simulink model "QuickModel"  (R2023b)
settings: Solver=VariableStepAuto  StartTime=0.0  StopTime=10.0  RelTol=1e-3
model workspace (MAT data in the model file):
  pqr = [0 0 0]
values from neighbouring files (symbols this model uses):
  alpha1 = 2.6    [QuickModel.m]    (also in QuickModelCode.m)
  alphadot = 0    [QuickModel.m]    (also in QuickModelCode.m)
  c_D_1 = .030    (= 0.03)    [QuickModel.m]    (also in QuickModelCode.m)
  c_D_alpha = ((2*c_L_1)/(pi*AR*e))*c_L_alpha    [QuickModel.m]    (also in QuickModelCode.m)
  c_D_delta_E = 0    [QuickModel.m]    (also in QuickModelCode.m)
  c_D_q = 0    [QuickModel.m]    (also in QuickModelCode.m)
  c_D_u = 0    [QuickModel.m]    (also in QuickModelCode.m)
  c_L_1 = .26    (= 0.26)    [QuickModel.m]    (also in QuickModelCode.m)
  c_L_alpha = c_L_alpha_W_mach + c_L_alpha_H    [QuickModel.m]    (also in QuickModelCode.m)
  c_L_alphadot = 2*c_L_alpha_H_mach*eta_H*(S_H/S_ft2)*(xbar_AC_H - xbar_CG)*(d_epsilon_dalpha_mach)    [QuickModel.m]    (also in QuickModelCode.m)
  c_L_delta_E = 0    [QuickModel.m]    (also in QuickModelCode.m)
  c_L_i_H = c_L_alpha_H_mach*eta_H*(S_H/S_ft2)    [QuickModel.m]    (also in QuickModelCode.m)
  c_L_q = piece1+piece2+piece3    [QuickModel.m]    (also in QuickModelCode.m)
  c_L_u = ((Mach^2)/(1-Mach^2))*c_L_1    (= 1.10842105263)    [QuickModel.m]    (also in QuickModelCode.m)
  c_m_1 = 0    [QuickModel.m]    (also in QuickModelCode.m)
  c_m_alpha = (c_L_alpha_W_mach*(xbar_CG - xbar_AC_WB)) - c_L_alpha_H_mach*eta_H*(S_H/S_ft2)*(1-d_epsilon_dalpha_mach)*(xbar_AC_H - xbar_CG)    [QuickModel.m]    (also in QuickModelCode.m)
  c_m_alphadot = -2*c_L_alpha_H_mach*eta_H*(S_H/S_ft2)*((xbar_AC_H - xbar_CG)^2)*d_epsilon_dalpha_mach    [QuickModel.m]    (also in QuickModelCode.m)
  c_m_delta_E = c_m_i_H * tau_E    [QuickModel.m]    (also in QuickModelCode.m)
  c_m_i_H = -c_L_alpha_H_mach*eta_H*(S_H/S_ft2) * (xbar_AC_H - xbar_CG)    [QuickModel.m]    (also in QuickModelCode.m)
  c_m_q = (frac * secondpiece * thirdpiece) + fourthpiece    [QuickModel.m]    (also in QuickModelCode.m)
  cbar_ft = 16.0    (= 16)    [QuickModel.m]    (also in QuickModelCode.m)
  deltaA = 0    [QuickModel.m]    (also in QuickModelCode.m)
  deltaE = 0    [QuickModel.m]    (also in QuickModelCode.m)
  i_H = 0    [QuickModel.m]    (also in QuickModelCode.m)
  qbar1 = 283.2    [QuickModel.m]    (also in QuickModelCode.m)
  S_ft2 = 530    [QuickModel.m]    (also in QuickModelCode.m)
  uv = a*Mach    (= 871.2)    [QuickModel.m]    (also in QuickModelCode.m)
  V_P_1 = 0    [QuickModel.m]    (also in QuickModelCode.m)
undefined symbols (not defined in the file or in its folder): c_D_i_H, c_m_u, delta_Stabilitator
libraries: shared6dof x1
settings Model: Creator=Owner  LastModifiedBy=Owner

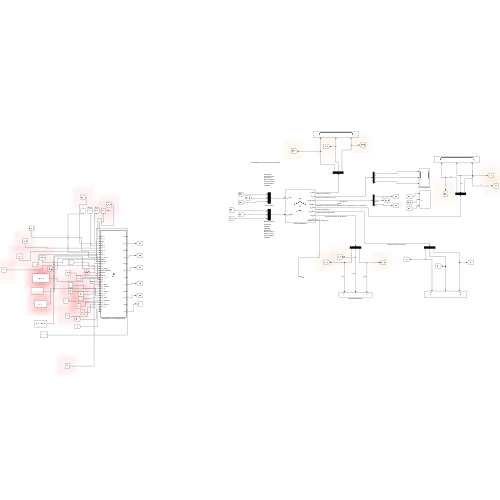
[thumbnail: Simulink's stored preview of the top-level diagram]
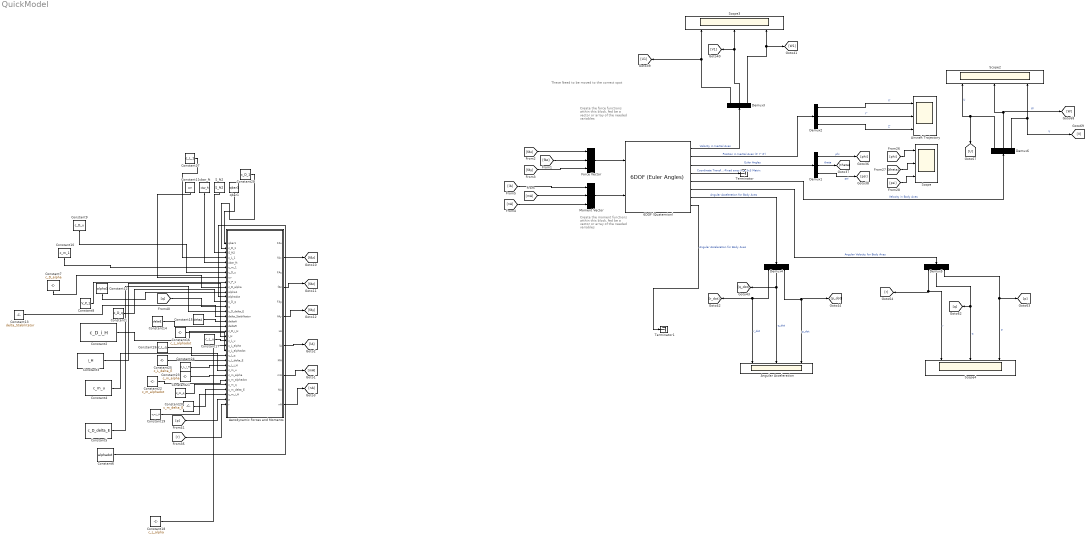
== system QuickModel ==
  note: These Need to be moved to the correct spot
  note: Create the moment functions within this block, fed be a vector or array of the needed variables
  note: Create the force functions within this block, fed be a vector or array of the needed variables
  6DOF (Quaternion) : shared6dof/6DOF (Euler Angles)  units=English (Velocity in ft/s)  mtype=Fixed  rep=Quaternion  xme_0=InitialInertialPosition  Vm_0=InitialVelocity  eul_0=InitialEulerOrientation  pm_0=pqr  mass_0=1.0  mass_e=0.5  mass_f=2.0  inertia=eye(3)  inertia_e=eye(3)  inertia_f=2*eye(3)  k_quat=1.0  vre_flag=on  abi_flag=off  aMode=0  xme_statename=''  Vm_statename=''  eul_statename=''  quat_statename=''  pm_statename=''  mass_statename=''
      settings: LibrarySourceBlock=aerolib6dof2/6DOF (Quaternion)
  Aerodynamic Forces and Moments : MATLAB Function  TreatAsAtomicUnit=on
  Aircraft Trajectory : Scope  NumInputPorts=3
  Angular Acceleration : Scope  NumInputPorts=3
  Constant1 : Constant  Value=c_D_q
  Constant10 : Constant  Value=c_m_1
  Constant11 : Constant  Value=uv
  Constant12 : Constant  Value=alpha1
  Constant13 : Constant  Value=delta_Stabilitator
  Constant14 : Constant  Value=deltaE
  Constant15 : Constant  Value=deltaA
  Constant16 : Constant  Value=c_L_alphadot
  Constant17 : Constant  Value=c_L_u
  Constant18 : Constant  Value=c_L_alpha
  Constant19 : Constant  Value=c_m_i_H
  Constant2 : Constant  Value=c_D_i_H
  Constant20 : Constant  Value=c_m_delta_E
  Constant21 : Constant  Value=c_m_q
  Constant22 : Constant  Value=c_m_alphadot
  Constant23 : Constant  Value=c_m_alpha
  Constant24 : Constant  Value=c_L_i_H
  Constant25 : Constant  Value=c_L_delta_E
  Constant26 : Constant  Value=c_L_q
  Constant27 : Constant  Value=c_L_1
  Constant28 : Constant  Value=c_D_1
  Constant3 : Constant  Value=i_H
  Constant4 : Constant  Value=c_m_u
  Constant5 : Constant  Value=c_D_delta_E
  Constant6 : Constant  Value=alphadot
  Constant7 : Constant  Value=c_D_alpha
  Constant8 : Constant  Value=V_P_1
  Constant9 : Constant  Value=c_D_u
  Demux{1..6} (6 alike) : Demux  Outputs=3
  Force Vector : Mux  Inputs=3
  Moment Vector : Mux  Inputs=3
  S_ft2 : Constant  Value=S_ft2
  Scope{,2..4} (4 alike) : Scope  NumInputPorts=3
  Terminator : Terminator
  Terminator1 : Terminator
  cbar_ft : Constant  Value=cbar_ft
  qbar1 : Constant  Value=qbar1
  wires:
  Demux1/1 -> [phi]  "phi"
  Demux4/3 -> [p_dot], Angular Acceleration/3  "p_dot"
  Demux1/2 -> [theta]  "theta"
  Demux6/2 -> [W], Scope2/2  "W"
  Demux6/3 -> [V], Scope2/3  "V"
  [fAy] -> Force Vector/3
  Demux4/1 -> [r_dot], Angular Acceleration/1  "r_dot"
  [lA] -> Moment Vector/1
  Demux4/2 -> [q_dot], Angular Acceleration/2  "q_dot"
  Demux5/2 -> [q], Scope4/2  "q"
  Demux5/3 -> [p], Scope4/3  "p"
  Demux5/1 -> [r], Scope4/1  "r"
  Demux3/3 -> Scope3/3, [W1]
  [phi] -> Scope/1
  [theta] -> Scope/2
  Demux3/1 -> Scope3/1, [U1]
  Demux2/2 -> Aircraft Trajectory/2  "Y'"
  Force Vector/1 -> 6DOF (Quaternion)/1
  Demux6/1 -> Scope2/1, [U]  "U"
  [nA] -> Moment Vector/3
  [fAz] -> Force Vector/2
  [fAx] -> Force Vector/1
  [mA] -> Moment Vector/2
  Demux2/3 -> Aircraft Trajectory/3  "Z'"
  6DOF (Quaternion)/7 -> Demux4/1  "Angular Acceleration for Body Axes"
  Moment Vector/1 -> 6DOF (Quaternion)/2
  Demux2/1 -> Aircraft Trajectory/1  "X'"
  6DOF (Quaternion)/1 -> Demux3/1  "Velocity in Inertial Axes"
  Demux3/2 -> [V1], Scope3/2
  Demux1/3 -> [psi]  "psi"
  [psi] -> Scope/3
  6DOF (Quaternion)/6 -> Demux5/1  "Angular Velocity for Body Axes"
  6DOF (Quaternion)/2 -> Demux2/1  "Position in Inertial Axes (X' Y' Z')"
  6DOF (Quaternion)/5 -> Demux6/1  "Velocity in Body Axes"
  6DOF (Quaternion)/3 -> Demux1/1  "Euler Angles"
  6DOF (Quaternion)/8 -> Terminator1/1  "Angular Acceleration for Body Axes"
  6DOF (Quaternion)/4 -> Terminator/1  "Coordinate Transformation from Flat Earth axes to Body-Fixed axes in a 3x3 Matrix"
  Constant25/1 -> Aerodynamic Forces and Moments/25(c_L_delta_E)
  Constant17/1 -> Aerodynamic Forces and Moments/21(c_L_u)
  Aerodynamic Forces and Moments/4(fAz) -> [fAz]
  [p] -> Aerodynamic Forces and Moments/33(p)
  Constant28/1 -> Aerodynamic Forces and Moments/2(c_D_1)
  Constant27/1 -> Aerodynamic Forces and Moments/4(c_L_1)
  Constant12/1 -> Aerodynamic Forces and Moments/11(alpha1)
  [r] -> Aerodynamic Forces and Moments/34(r)
  Constant7/1 -> Aerodynamic Forces and Moments/10(c_D_alpha)
  Constant10/1 -> Aerodynamic Forces and Moments/6(c_m_1)
  Constant14/1 -> Aerodynamic Forces and Moments/18(deltaR)
  Constant26/1 -> Aerodynamic Forces and Moments/24(c_L_q)
  [q] -> Aerodynamic Forces and Moments/14(q)
  Constant9/1 -> Aerodynamic Forces and Moments/7(c_D_u)
  Constant20/1 -> Aerodynamic Forces and Moments/31(c_m_delta_E)
  Constant15/1 -> Aerodynamic Forces and Moments/17(deltaA)
  Constant13/1 -> Aerodynamic Forces and Moments/16(delta_Stabilitator)
  Aerodynamic Forces and Moments/12(nA) -> [nA]
  Aerodynamic Forces and Moments/6(fAy) -> [fAy]
  Aerodynamic Forces and Moments/10(mA) -> [mA]
  Constant21/1 -> Aerodynamic Forces and Moments/30(c_m_q)
  Constant11/1 -> Aerodynamic Forces and Moments/8(uv)
  Constant19/1 -> Aerodynamic Forces and Moments/32(c_m_i_H)
  qbar1/1 -> Aerodynamic Forces and Moments/1(qbar1)
  Aerodynamic Forces and Moments/8(lA) -> [lA]
  cbar_ft/1 -> Aerodynamic Forces and Moments/5(cbar_ft)
  Constant16/1 -> Aerodynamic Forces and Moments/23(c_L_alphadot)
  Constant18/1 -> Aerodynamic Forces and Moments/22(c_L_alpha)
  Aerodynamic Forces and Moments/2(fAx) -> [fAx]
  Constant22/1 -> Aerodynamic Forces and Moments/29(c_m_alphadot)
  Constant24/1 -> Aerodynamic Forces and Moments/26(c_L_i_H)
  Constant23/1 -> Aerodynamic Forces and Moments/28(c_m_alpha)
  S_ft2/1 -> Aerodynamic Forces and Moments/3(S_ft2)
  Constant1/1 -> Aerodynamic Forces and Moments/13(c_D_q)
  Constant2/1 -> Aerodynamic Forces and Moments/19(c_D_i_H)
  Constant3/1 -> Aerodynamic Forces and Moments/20(i_H)
  Constant4/1 -> Aerodynamic Forces and Moments/27(c_m_u)
  Constant5/1 -> Aerodynamic Forces and Moments/15(c_D_delta_E)
  Constant6/1 -> Aerodynamic Forces and Moments/12(alphadot)
  Constant8/1 -> Aerodynamic Forces and Moments/9(V_P_1)

== matlab function QuickModel/Aerodynamic Forces and Moments ==
  data: qbar1 input; c_D_1 input; S_ft2 input; c_L_1 input; cbar_ft input; c_m_1 input; c_D_u input; uv input; FAx output; V_P_1 input; c_D_alpha input; alpha1 input; alphadot input; c_D_q input; q input; c_D_delta_E input; delta_Stabilitator input; deltaA input; deltaR input; c_D_i_H input; i_H input; c_L_u input; c_L_alpha input; c_L_alphadot input; c_L_q input; c_L_delta_E input; c_L_i_H input; c_m_u input; c_m_alpha input; c_m_alphadot input; c_m_q input; c_m_delta_E input; c_m_i_H input; fAx output; FAz output; fAz output; FAy output; fAy output; LA output; lA output; MA output; mA output; NA output; nA output; p input; r input
function [FAx, fAx, FAz, fAz, FAy, fAy, LA, lA, MA, mA, NA, nA]  = fcn(qbar1, c_D_1, S_ft2, c_L_1, cbar_ft, c_m_1, c_D_u, uv, V_P_1, c_D_alpha, alpha1, alphadot, c_D_q, q, c_D_delta_E, delta_Stabilitator, deltaA, deltaR, c_D_i_H, i_H, c_L_u, c_L_alpha, c_L_alphadot, c_L_q, c_L_delta_E, c_L_i_H, c_m_u, c_m_alpha, c_m_alphadot, c_m_q, c_m_delta_E, c_m_i_H, p, r)

FAx = -qbar1*S_ft2*c_D_1;
fAx = (qbar1*S_ft2)*(((-(c_D_u+(2*c_D_1)))*(uv/V_P_1)) + ((c_D_alpha + c_L_1)*(alpha1)) - c_D_alphadot*((alphadot*cbar_ft)/(2*V_P_1)) - c_D_q*((q*cbar)/(2*V_P_1)) - (c_D_delta_E*delta_Stabilitator)-(c_D_i_H*i_H));

FAz = -qbar1*S_ft2*c_L_1;
fAz = (qbar1*S_ft2)*(((-(c_L_u+(2*c_L_1)))*(uv/V_P_1)) + ((c_L_alpha + c_D_1)*(alpha1)) - c_L_alphadot*((alphadot*cbar_ft)/(2*V_P_1)) - c_L_q*((q*cbar)/(2*V_P_1)) - (c_L_delta_E*delta_Stabilitator)-(c_L_i_H*i_H));

FAy = -qbar1*S_ft2*c_Y_1;
fAy = -qbar1*S_ft2 * ((c_Y_beta*beta) + c_Y_betadot * ((betadot*b_ft)/(2*V_P_1)) + c_Y_p*((p*b_ft)/(2*V_P_1)) + c_Y_r * ((r*b_ft)/(2*V_P_1)) +(c_Y_delta_A * deltaA) + (c_Y_delta_R*deltaR));

LA = -qbar1*S_ft2*b_ft*c_l_1;
lA = -qbar1*S_ft2*b_ft*((c_l_beta*beta) + c_l_betadot * ((betadot*b_ft)/(2*V_P_1)) + c_l_p*((p*b_ft)/(2*V_P_1)) + c_l_r * ((r*b_ft)/(2*V_P_1)) +(c_l_delta_A * deltaA) + (c_l_delta_R*deltaR));

MA = -qbar1*S_ft2*cbar_ft*c_m_1;
mA = (qbar1*S_ft2*cbar_ft)*(((-(c_m_u+(2*c_m_1)))*(uv/V_P_1)) + (c_m_alpha*alpha1) + c_m_alphadot*((alphadot*cbar_ft)/(2*V_P_1)) + c_m_q*((q*cbar_ft)/(2*V_P_1)) + (c_m_delta_E*delta_Stabilitator)+(c_L_i_H*i_H));

NA = -qbar1*S_ft2*b_ft*c_n_1;
nA = -qbar1*S_ft2*b_ft*((c_n_beta*beta) + c_n_betadot * ((betadot*b_ft)/(2*V_P_1)) + c_n_p*((p*b_ft)/(2*V_P_1)) + c_n_r * ((r*b_ft)/(2*V_P_1)) +(c_n_delta_A * deltaA) + (c_n_delta_R*deltaR));

%Need to get rid of fAy and lA and nA, leave MA and mA
